simulink model "eq_analysis_1"  (R2017b)
settings: Solver=VariableStepAuto  StartTime=0.0  StopTime=10.0  RelTol=1e-3
values from neighbouring files (symbols this model uses):
  Ac = [0 1;-wn(i)^2 -2*dmp(index)*wn(i)]    [hw8_plus.m]
  Bc = [0; -1]    [hw8_plus.m]
  Cc = [1 0;[-wn(i)^2 -2*dmp(index)*wn(i)]]    [hw8_plus.m]
  Dc = [0;0]    [hw8_plus.m]
  dt = tt_acc(2,1)-tt_acc(1,1)    [hw8_plus.m]
settings Model: Creator=skyran  LastModifiedBy=skyran

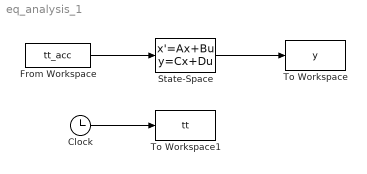
== system eq_analysis_1 ==
  Clock : Clock
  From Workspace : FromWorkspace  VariableName=tt_acc  SampleTime=dt  OutputAfterFinalValue=Setting to zero
  State-Space : StateSpace  A=Ac  B=Bc  C=Cc  D=Dc  InitialCondition=0
  To Workspace : ToWorkspace  VariableName=y  SaveFormat=Timeseries  SampleTime=-1
  To Workspace1 : ToWorkspace  VariableName=tt  SaveFormat=Timeseries  SampleTime=-1
  wires:
  From Workspace/1 -> State-Space/1
  State-Space/1 -> To Workspace/1
  Clock/1 -> To Workspace1/1
